simulink model "untitled2"  (R2024b)
settings: Solver=FixedStepAuto  StartTime=0.0  StopTime=inf  FixedStep=0.01  RelTol=1e-3  EnableMultiTasking=on
undefined symbols (not defined in the file or in its folder): qbreak
libraries: simulink x70, arduinolib x31, dspswit3 x9, dspstat3 x4, arduinosensorlib x2, dspfdesign x2
(part 1 of 3)
settings Model: ExtModeTrigDuration=2  Creator=ARIES  LastModifiedBy=ARIES
settings SolverCC: AutoInsertRateTranBlk=on
settings OptimizationCC: EnhancedBackFolding=on  PassReuseOutputArgsAs=Individual arguments  ZeroExternalMemoryAtStartup=off  ZeroInternalMemoryAtStartup=off  MaxStackSize=64  OptimizeBlockOrder=speed  DifferentSizesBufferReuse=on  OptimizationCustomize=off  EfficientTunableParamExpr=on
settings DebuggingCC: ParameterTunabilityLossMsg=error
settings HardwareCC: ProdBitPerPointer=32  ProdBitPerSizeT=32  ProdBitPerPtrDiffT=32  ProdLargestAtomicInteger=Long  ProdLargestAtomicFloat=Double  ProdWordSize=32  ProdHWDeviceType=ARM Compatible->ARM Cortex
settings SFSimCC: MATLABDynamicMemAlloc=off
settings RTWCC: Description=Embedded Coder  SystemTargetFile=ert.tlc  HardwareBoard=Arduino MKR WiFi 1010  TemplateMakefile=ert_default_tmf  Toolchain=Arduino ARM  BuildConfiguration=Faster Runs
settings CodeAppCC: ForceParamTrailComments=on  IgnoreCustomStorageClasses=off  OperatorAnnotations=on  SimulinkDataObjDesc=on  SFDataObjDesc=on  InsertBlockDesc=on
settings ERTTargetCC: SupportContinuousTime=on  SupportVariableSizeSignals=on  ExtModeTransport=3  ExtModeStaticAlloc=on  ExtModeAutomaticAllocSize=off  ExtModeStaticAllocSize=8192  ExtModeMexFile=ext_xcp  ExtModeIntrfLevel=Level2 - Open  InlinedParameterPlacement=Hierarchical

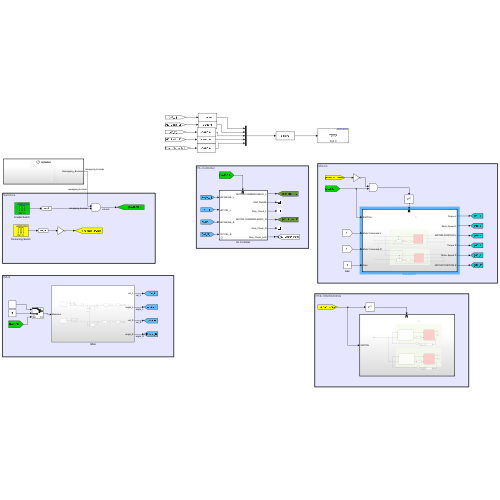
[thumbnail: Simulink's stored preview of the top-level diagram]
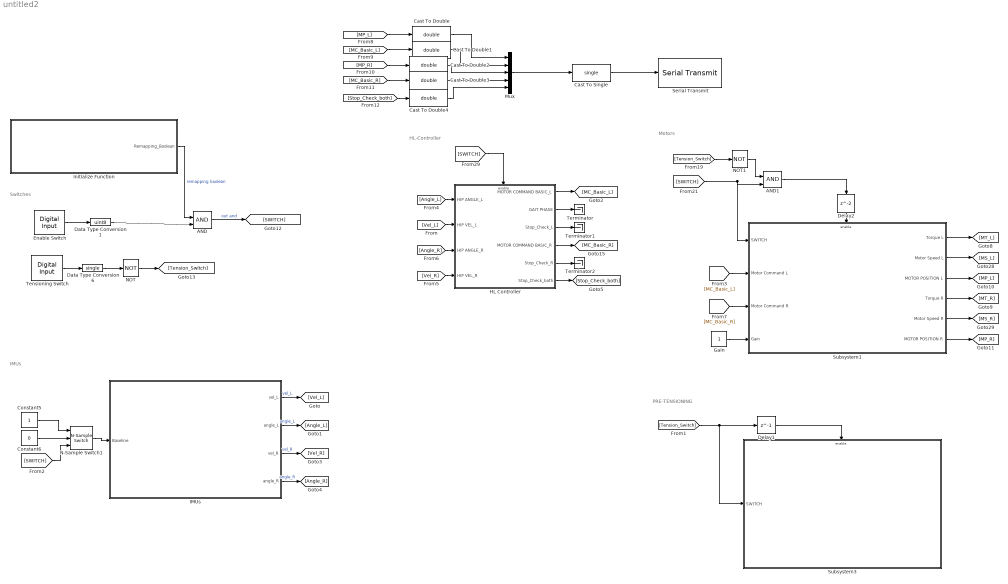
== system untitled2 ==
  note: PRE-TENSIONING
  note: Switches
  note: HL-Controller
  note: IMUs
  note: Motors
  AND : Logic  IconShape=distinctive  AllPortsSameDT=off  OutDataTypeStr=boolean
  AND1 : Logic  IconShape=distinctive  AllPortsSameDT=off  OutDataTypeStr=boolean
  Cast To Double{,1..4} (5 alike) : DataTypeConversion  OutDataTypeStr=double  SaturateOnIntegerOverflow=off  RndMeth=Floor
  Cast To Single : DataTypeConversion  OutDataTypeStr=single  SaturateOnIntegerOverflow=off  RndMeth=Floor
  Constant5 : Constant
  Constant6 : Constant  Value=0
  Data Type Conversion1 : DataTypeConversion  OutDataTypeStr=uint8  SaturateOnIntegerOverflow=off  RndMeth=Floor
  Data Type Conversion6 : DataTypeConversion  OutDataTypeStr=single  SaturateOnIntegerOverflow=off  RndMeth=Floor
  Delay1 : Delay  DelayLength=1
  Delay2 : Delay
  Enable Switch : arduinolib/Digital Input  pinNumber=6  mode=Default  Direction=input  SampleTime=0.01  blockPlatform=arduino
      settings: SourceProductName=Common
  Gain : Constant
  HL Controller : Subsystem  mask{LAG=pi/7, THR=5, AMPL=-6.5}
      mask prompts: LAG "Lag compensation (rad)"; THR "Stop Threshold"; AMPL "Motor position desired amplitude"
  IMUs : Subsystem
  Initialize Function : Subsystem  TreatAsAtomicUnit=on
  Mux : Mux  Inputs=5
  N-Sample Switch1 : dspswit3/N-Sample Switch  N=10  reset=on  TriggerType=Rising edge  Ts=0.01
  NOT : Logic  Operator=NOT  IconShape=distinctive  AllPortsSameDT=off  OutDataTypeStr=boolean
  NOT1 : Logic  Operator=NOT  IconShape=distinctive  AllPortsSameDT=off  OutDataTypeStr=boolean
  Serial Transmit : arduinolib/Serial Transmit  portNumber=0  sendmode=write  sendformat=Decimal  floatprecision=2  header=[]  terminator=[]  blockPlatform=ARDUINO
      settings: SourceProductName=Common
  Subsystem1 : Subsystem
  Subsystem3 : Subsystem
  Tensioning Switch : arduinolib/Digital Input  pinNumber=5  mode=Input Pullup  Direction=input  SampleTime=0.01  blockPlatform=arduino
      settings: SourceProductName=Common
  Terminator : Terminator
  Terminator1 : Terminator
  Terminator2 : Terminator
  wires:
  Subsystem1/1(Torque L) -> [MT_L]
  AND/1 -> [SWITCH]  "out and"
  [Tension_Switch] -> NOT1/1
  IMUs/4(angle_R) -> [Angle_R]  "angle_R"
  Tensioning Switch/1 -> Data Type Conversion6/1
  Subsystem1/6(MOTOR POSITION R) -> [MP_R]
  Constant5/1 -> N-Sample Switch1/1
  [Tension_Switch] -> Subsystem3/1(SWITCH), Delay1/1
  IMUs/3(vel_R) -> [Vel_R]  "vel_R"
  AND1/1 -> Delay2/1
  NOT1/1 -> AND1/1
  Subsystem1/3(MOTOR POSITION L) -> [MP_L]
  Data Type Conversion6/1 -> NOT/1
  [Vel_R] -> HL Controller/4(HIP VEL_R)
  HL Controller/1(MOTOR COMMAND BASIC_L) -> [MC_Basic_L]
  Delay2/1 -> Subsystem1/Enable
  HL Controller/4(MOTOR COMMAND BASIC_R) -> [MC_Basic_R]
  Enable Switch/1 -> Data Type Conversion1/1
  IMUs/2(angle_L) -> [Angle_L]  "angle_L"
  Subsystem1/5(Motor Speed R) -> [MS_R]
  Data Type Conversion1/1 -> AND/2
  N-Sample Switch1/1 -> IMUs/1(Baseline)
  Delay1/1 -> Subsystem3/Enable
  NOT/1 -> [Tension_Switch]
  Constant6/1 -> N-Sample Switch1/2
  [Angle_R] -> HL Controller/3(HIP ANGLE_R)
  Subsystem1/2(Motor Speed L) -> [MS_L]
  [SWITCH] -> HL Controller/Enable
  Initialize Function/1(Remapping_Boolean) -> AND/1  "remapping boolean"
  [MC_Basic_R] -> Subsystem1/3(Motor Command R)
  [SWITCH] -> N-Sample Switch1/3
  [Angle_L] -> HL Controller/1(HIP ANGLE_L)
  [Vel_L] -> HL Controller/2(HIP VEL_L)
  IMUs/1(vel_L) -> [Vel_L]  "vel_L"
  [SWITCH] -> AND1/2, Subsystem1/1(SWITCH)
  Subsystem1/4(Torque R) -> [MT_R]
  [MC_Basic_L] -> Subsystem1/2(Motor Command L)
  Gain/1 -> Subsystem1/4(Gain)
  Mux/1 -> Cast To Single/1
  Cast To Single/1 -> Serial Transmit/1
  [MP_L] -> Cast To Double/1
  [MC_Basic_L] -> Cast To Double1/1
  [MP_R] -> Cast To Double2/1
  [MC_Basic_R] -> Cast To Double3/1
  HL Controller/6(Stop_Check_both) -> [Stop_Check_both]
  [Stop_Check_both] -> Cast To Double4/1
  HL Controller/5(Stop_Check_R) -> Terminator2/1
  HL Controller/3(Stop_Check_L) -> Terminator1/1
  HL Controller/2(GAIT PHASE) -> Terminator/1
  Cast To Double/1 -> Mux/1
  Cast To Double1/1 -> Mux/2
  Cast To Double3/1 -> Mux/4
  Cast To Double2/1 -> Mux/3
  Cast To Double4/1 -> Mux/5

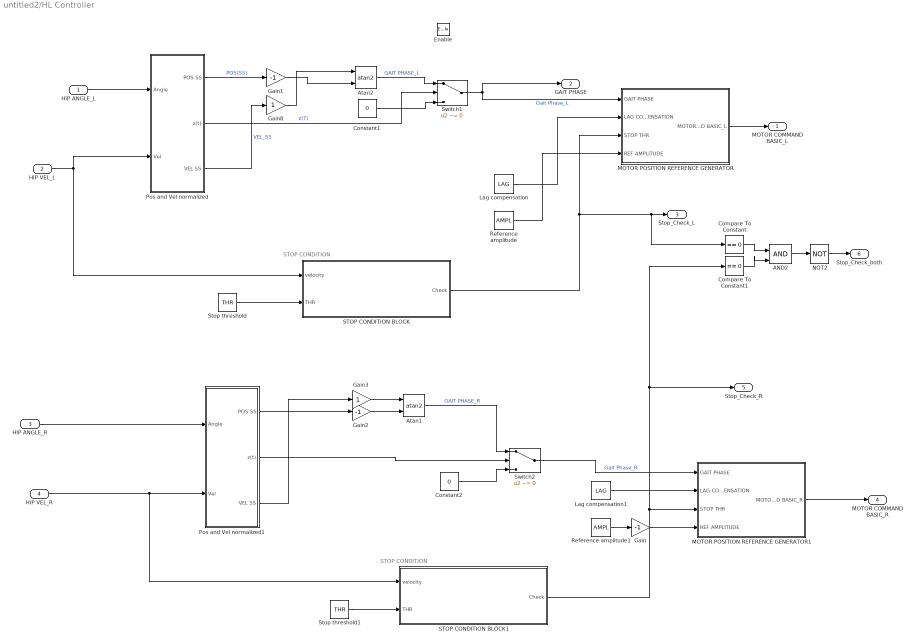
== system untitled2/HL Controller ==
  note: STOP CONDITION
  note: STOP CONDITION
  HIP ANGLE_L : Inport
  HIP VEL_L : Inport  Port=2
  HIP ANGLE_R : Inport  Port=3
  HIP VEL_R : Inport  Port=4
  Enable : EnablePort
  AND2 : Logic  IconShape=distinctive  AllPortsSameDT=off  OutDataTypeStr=boolean
  Atan1 : Trigonometry  Operator=atan2
  Atan2 : Trigonometry  Operator=atan2
  Compare To Constant : simulink/Logic and Bit Operations/Compare To Constant  relop===  const=0  OutDataTypeStr=boolean
  Compare To Constant1 : simulink/Logic and Bit Operations/Compare To Constant  relop===  const=0  OutDataTypeStr=boolean
  Constant1 : Constant  Value=0
  Constant2 : Constant  Value=0
  Gain : Gain  Gain=-1
  Gain1 : Gain  Gain=-1
  Gain2 : Gain  Gain=-1
  Gain3 : Gain
  Gain8 : Gain
  Lag compensation : Constant  Value=LAG
  Lag compensation1 : Constant  Value=LAG
  MOTOR POSITION REFERENCE GENERATOR : Subsystem
  MOTOR POSITION REFERENCE GENERATOR1 : Subsystem
  NOT2 : Logic  Operator=NOT  IconShape=distinctive  AllPortsSameDT=off  OutDataTypeStr=boolean
  Pos and Vel normalized : Subsystem
  Pos and Vel normalized1 : Subsystem
  Reference amplitude : Constant  Value=AMPL
  Reference amplitude1 : Constant  Value=AMPL
  STOP CONDITION BLOCK : Subsystem
  STOP CONDITION BLOCK1 : Subsystem
  Stop threshold : Constant  Value=THR
  Stop threshold1 : Constant  Value=THR
  Switch1 : Switch  Criteria=u2 ~= 0  SaturateOnIntegerOverflow=off  InputSameDT=off
  Switch2 : Switch  Criteria=u2 ~= 0  SaturateOnIntegerOverflow=off  InputSameDT=off
  MOTOR COMMAND BASIC_L : Outport
  GAIT PHASE : Outport  Port=2
  Stop_Check_L : Outport  Port=3
  MOTOR COMMAND BASIC_R : Outport  Port=4
  Stop_Check_R : Outport  Port=5
  Stop_Check_both : Outport  Port=6
  wires:
  Gain8/1 -> Atan2/1
  Atan2/1 -> Switch1/1  "GAIT PHASE_L"
  Switch1/1 -> GAIT PHASE/1, MOTOR POSITION REFERENCE GENERATOR/1(GAIT PHASE)  "Gait Phase_L"
  Constant1/1 -> Switch1/3
  Gain1/1 -> Atan2/2
  Pos and Vel normalized/1(POS SS) -> Gain1/1  "POS(SS)"
  Pos and Vel normalized/2(z(t)) -> Switch1/2  "z(T)"
  Pos and Vel normalized/3(VEL SS) -> Gain8/1  "VEL_SS"
  HIP VEL_L/1 -> STOP CONDITION BLOCK/1(velocity), Pos and Vel normalized/2(Vel)
  HIP ANGLE_L/1 -> Pos and Vel normalized/1(Angle)
  Lag compensation/1 -> MOTOR POSITION REFERENCE GENERATOR/2(LAG COMPENSATION)
  Stop threshold/1 -> STOP CONDITION BLOCK/2(THR)
  Reference amplitude/1 -> MOTOR POSITION REFERENCE GENERATOR/4(REF AMPLITUDE)
  MOTOR POSITION REFERENCE GENERATOR/1(MOTOR COMMAND BASIC_L) -> MOTOR COMMAND BASIC_L/1
  Switch2/1 -> MOTOR POSITION REFERENCE GENERATOR1/1(GAIT PHASE)  "Gait Phase_R"
  Lag compensation1/1 -> MOTOR POSITION REFERENCE GENERATOR1/2(LAG COMPENSATION)
  Stop threshold1/1 -> STOP CONDITION BLOCK1/2(THR)
  Pos and Vel normalized1/2(z(t)) -> Switch2/2
  Pos and Vel normalized1/1(POS SS) -> Gain2/1
  Gain2/1 -> Atan1/2
  Constant2/1 -> Switch2/3
  Gain3/1 -> Atan1/1
  Pos and Vel normalized1/3(VEL SS) -> Gain3/1
  Atan1/1 -> Switch2/1  "GAIT PHASE_R"
  HIP ANGLE_R/1 -> Pos and Vel normalized1/1(Angle)
  MOTOR POSITION REFERENCE GENERATOR1/1(MOTOR COMMAND BASIC_R) -> MOTOR COMMAND BASIC_R/1
  HIP VEL_R/1 -> STOP CONDITION BLOCK1/1(velocity), Pos and Vel normalized1/2(Vel)
  Reference amplitude1/1 -> Gain/1
  Compare To Constant1/1 -> AND2/2
  NOT2/1 -> Stop_Check_both/1
  AND2/1 -> NOT2/1
  STOP CONDITION BLOCK1/1(Check) -> MOTOR POSITION REFERENCE GENERATOR1/3(STOP THR), Stop_Check_R/1, Compare To Constant1/1
  Compare To Constant/1 -> AND2/1
  STOP CONDITION BLOCK/1(Check) -> MOTOR POSITION REFERENCE GENERATOR/3(STOP THR), Stop_Check_L/1, Compare To Constant/1
  Gain/1 -> MOTOR POSITION REFERENCE GENERATOR1/4(REF AMPLITUDE)

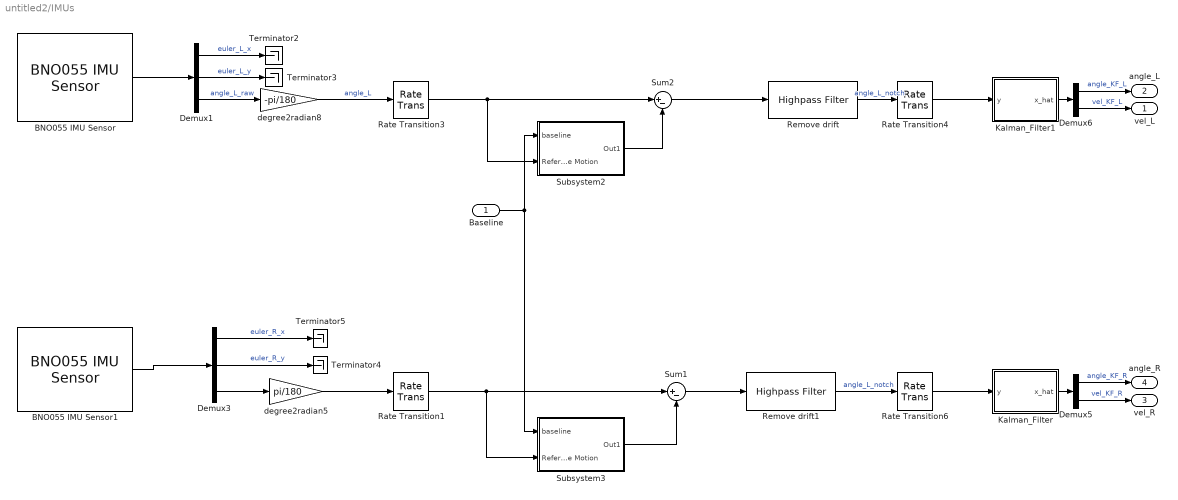
== system untitled2/IMUs ==
  Baseline : Inport
  BNO055 IMU Sensor : arduinosensorlib/BNO055 IMU Sensor  I2CModule=0  SlaveAddress=0x28  OperationMode=Fusion  Accel=off  AngularRate=off  MagField=off  EulerAngles=on  Quat=off  LinearAccel=off  GravityVector=off  Status=off  Timestamp=off  AccelRange=4G  AccelBW=62.5 Hz  GyroRange=2000 dps  GyroBW=32 Hz  MagODR=10 Hz  spf=1  SampleTime=-1  blockPlatform=ARDUINO  QueueSizeFactor=1
      settings: SourceProductName=Sensors
  BNO055 IMU Sensor1 : arduinosensorlib/BNO055 IMU Sensor  I2CModule=0  SlaveAddress=0x29  OperationMode=Fusion  Accel=off  AngularRate=off  MagField=off  EulerAngles=on  Quat=off  LinearAccel=off  GravityVector=off  Status=off  Timestamp=off  AccelRange=4G  AccelBW=62.5 Hz  GyroRange=2000 dps  GyroBW=32 Hz  MagODR=10 Hz  spf=1  SampleTime=-1  blockPlatform=ARDUINO  QueueSizeFactor=1
      settings: SourceProductName=Sensors
  Demux1 : Demux  Outputs=3
  Demux3 : Demux  Outputs=3
  Demux5 : Demux  Outputs=2
  Demux6 : Demux  Outputs=2
  Kalman_Filter : MATLAB Function  TreatAsAtomicUnit=on
  Kalman_Filter1 : MATLAB Function  TreatAsAtomicUnit=on
  Rate Transition{1,3..4,6} (4 alike) : RateTransition  OutPortSampleTime=0.01
  Remove drift : dspfdesign/Highpass Filter  FilterType=IIR  DesignForMinimumOrder=off  FilterOrder=2  StopbandFrequency=8e3  PassbandFrequency=0.1  StopbandAttenuation=40  PassbandRipple=0.1  SampleRateMode=Specify on dialog  SampleRate=100  SimulateUsing=Interpreted execution  roundingMode=Floor  coeffsDataTypeStr=fixdt(1,16)
  Remove drift1 : dspfdesign/Highpass Filter  FilterType=IIR  DesignForMinimumOrder=off  FilterOrder=2  StopbandFrequency=8e3  PassbandFrequency=0.1  StopbandAttenuation=40  PassbandRipple=0.1  SampleRateMode=Specify on dialog  SampleRate=100  SimulateUsing=Interpreted execution  roundingMode=Floor  coeffsDataTypeStr=fixdt(1,16)
  Subsystem2 : Subsystem
  Subsystem3 : Subsystem
  Sum1 : Sum  Inputs=|+-
  Sum2 : Sum  Inputs=|+-
  Terminator{2..5} (4 alike) : Terminator
  degree2radian5 : Gain  Gain=pi/180
  degree2radian8 : Gain  Gain=-pi/180
  vel_L : Outport
  angle_L : Outport  Port=2
  vel_R : Outport  Port=3
  angle_R : Outport  Port=4
  wires:
  BNO055 IMU Sensor/1 -> Demux1/1
  BNO055 IMU Sensor1/1 -> Demux3/1
  Demux1/1 -> Terminator2/1  "euler_L_x"
  Demux1/3 -> degree2radian8/1  "angle_L_raw"
  Demux1/2 -> Terminator3/1  "euler_L_y"
  Demux3/1 -> Terminator5/1  "euler_R_x"
  Demux3/2 -> Terminator4/1  "euler_R_y"
  Demux3/3 -> degree2radian5/1
  Remove drift/1 -> Rate Transition4/1  "angle_L_notch"
  Remove drift1/1 -> Rate Transition6/1  "angle_L_notch"
  Kalman_Filter/1(x_hat) -> Demux5/1
  Demux5/1 -> angle_R/1  "angle_KF_R"
  Demux5/2 -> vel_R/1  "vel_KF_R"
  Sum2/1 -> Remove drift/1
  Rate Transition3/1 -> Subsystem2/2(Reference Motion), Sum2/1
  Baseline/1 -> Subsystem2/1(baseline), Subsystem3/1(baseline)
  Subsystem2/1(Out1) -> Sum2/2
  Rate Transition1/1 -> Subsystem3/2(Reference Motion), Sum1/1
  Subsystem3/1(Out1) -> Sum1/2
  Sum1/1 -> Remove drift1/1
  degree2radian8/1 -> Rate Transition3/1  "angle_L"
  degree2radian5/1 -> Rate Transition1/1
  Rate Transition6/1 -> Kalman_Filter/1(y)
  Demux6/1 -> angle_L/1  "angle_KF_L"
  Demux6/2 -> vel_L/1  "vel_KF_L"
  Kalman_Filter1/1(x_hat) -> Demux6/1
  Rate Transition4/1 -> Kalman_Filter1/1(y)

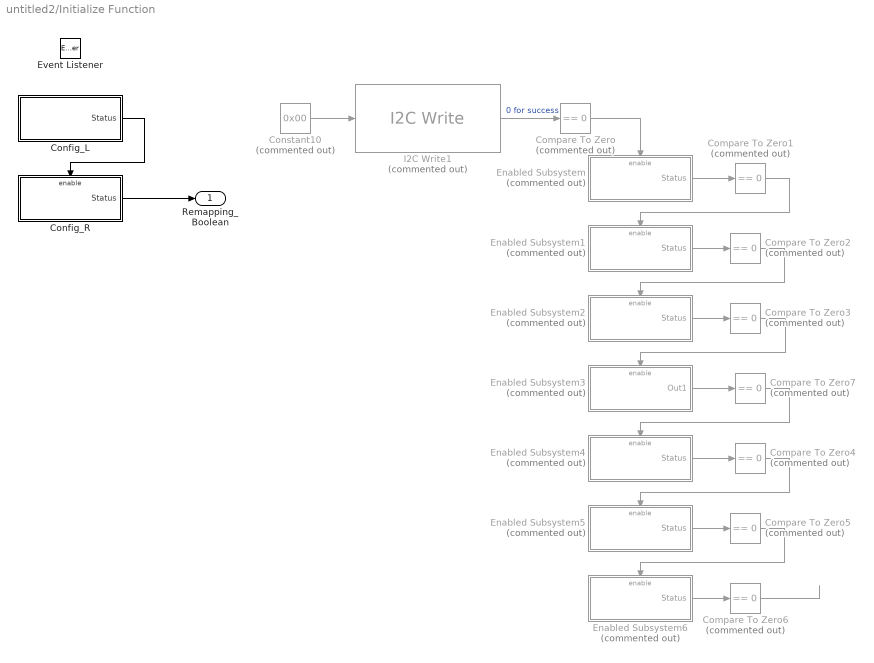
== system untitled2/Initialize Function ==
  Compare To Zero{,1..7} (8 alike) : simulink/Logic and Bit Operations/Compare To Zero  Commented=on  relop===  OutDataTypeStr=boolean
  "Config_L " : Subsystem  TreatAsAtomicUnit=on
  Config_R : Subsystem  TreatAsAtomicUnit=on
  Constant10 : Constant  Commented=on  Value=0x00
  Enabled Subsystem : Subsystem  Commented=on  TreatAsAtomicUnit=on
  Enabled Subsystem1 : Subsystem  Commented=on  TreatAsAtomicUnit=on
  Enabled Subsystem2 : Subsystem  Commented=on  TreatAsAtomicUnit=on
  Enabled Subsystem3 : Subsystem  Commented=on  TreatAsAtomicUnit=on
  Enabled Subsystem4 : Subsystem  Commented=on  TreatAsAtomicUnit=on
  Enabled Subsystem5 : Subsystem  Commented=on  TreatAsAtomicUnit=on
  Enabled Subsystem6 : Subsystem  Commented=on  TreatAsAtomicUnit=on
  Event Listener : EventListener  DisableCoverage=on  EventName=reset
  I2C Write1 : arduinolib/I2C Write  Commented=on  I2CModule=0  Mode=Master  SlaveAddress=0x29  SlaveByteOrder=BigEndian  Direction=Transmitter  RegisterAddressMode=on  RegisterAddress=0x3D  SlaveDataType=uint8  DataLength=1  NoAck=off  RepeatedStart=off  OutputStatus=on  blockPlatform=ARDUINO
      settings: SourceProductName=Common
  Remapping_Boolean : Outport
  wires:
  Compare To Zero/1 -> Enabled Subsystem/Enable
  I2C Write1/1 -> Compare To Zero/1  "0 for success"
  Constant10/1 -> I2C Write1/1
  Enabled Subsystem/1(Status) -> Compare To Zero1/1
  Compare To Zero1/1 -> Enabled Subsystem1/Enable
  Enabled Subsystem1/1(Status) -> Compare To Zero2/1
  Compare To Zero2/1 -> Enabled Subsystem2/Enable
  Enabled Subsystem2/1(Status) -> Compare To Zero3/1
  Compare To Zero3/1 -> Enabled Subsystem3/Enable
  Enabled Subsystem5/1(Status) -> Compare To Zero5/1
  Enabled Subsystem6/1(Status) -> Compare To Zero6/1
  Compare To Zero4/1 -> Enabled Subsystem5/Enable
  Enabled Subsystem4/1(Status) -> Compare To Zero4/1
  Compare To Zero5/1 -> Enabled Subsystem6/Enable
  Enabled Subsystem3/1(Out1) -> Compare To Zero7/1
  Compare To Zero7/1 -> Enabled Subsystem4/Enable
  Compare To Zero6/1 -> ?
  "Config_L "/1(Status) -> Config_R/Enable
  Config_R/1(Status) -> Remapping_Boolean/1

== system untitled2/Subsystem1 ==
  note: LeftLeg_AK60-6 Motor Modules
  note: RightLeg_AK60-6 Motor Modules
  SWITCH : Inport
  Motor Command L : Inport  Port=2
  Motor Command R : Inport  Port=3
  Gain : Inport  Port=4
  Enable : EnablePort  StatesWhenEnabling=reset
  Data Type Conversion1 : DataTypeConversion  OutDataTypeStr=single  SaturateOnIntegerOverflow=off  RndMeth=Floor
  Data Type Conversion2 : DataTypeConversion  OutDataTypeStr=single  SaturateOnIntegerOverflow=off  RndMeth=Floor
  Left Motor Velocity1 : Subsystem
  PID1 : Subsystem
  PID2 : Subsystem
  Product : Product
  Product1 : Product
  Right Motor Velocity1 : Subsystem
  Torque L : Outport
  Motor Speed L : Outport  Port=2
  MOTOR POSITION L : Outport  Port=3
  Torque R : Outport  Port=4
  Motor Speed R : Outport  Port=5
  MOTOR POSITION R : Outport  Port=6
  wires:
  Motor Command L/1 -> PID1/1(Ref)
  PID1/1(Velocity output) -> Product/1
  Left Motor Velocity1/1(MOTOR POSITION) -> PID1/2(Actual Motion), MOTOR POSITION L/1
  Data Type Conversion1/1 -> Left Motor Velocity1/2(Motor command)
  Motor Command R/1 -> PID2/1(Ref)
  PID2/1(Velocity output) -> Product1/2
  SWITCH/1 -> PID2/Enable, Right Motor Velocity1/1(SWITCH), Left Motor Velocity1/1(SWITCH), PID1/Enable
  Data Type Conversion2/1 -> Right Motor Velocity1/2(Motor command)
  Left Motor Velocity1/3(MOTOR TORQUE) -> Torque L/1
  Left Motor Velocity1/2(MOTOR SPEED) -> Motor Speed L/1
  Right Motor Velocity1/1(MOTOR POSITION) -> MOTOR POSITION R/1, PID2/2(Actual Motion)
  Right Motor Velocity1/2(MOTOR SPEED) -> Motor Speed R/1
  Right Motor Velocity1/3(MOTOR TORQUE) -> Torque R/1
  Product/1 -> Data Type Conversion1/1
  Product1/1 -> Data Type Conversion2/1
  Gain/1 -> Product1/1, Product/2

== system untitled2/Subsystem3 ==
  note: RightLeg_AK60-6 Motor Modules
  note: LeftLeg_AK60-6 Motor Modules
  SWITCH : Inport
  Enable : EnablePort  StatesWhenEnabling=reset
  Abs : Abs  SaturateOnIntegerOverflow=off
  Abs1 : Abs  SaturateOnIntegerOverflow=off
  Chart : Stateflow chart  TreatAsAtomicUnit=on
  Chart1 : Stateflow chart  TreatAsAtomicUnit=on
  Data Type Conversion1 : DataTypeConversion  OutDataTypeStr=single  SaturateOnIntegerOverflow=off  RndMeth=Floor
  Data Type Conversion6 : DataTypeConversion  OutDataTypeStr=single  SaturateOnIntegerOverflow=off  RndMeth=Floor
  Left Motor Velocity : Subsystem
  Right Motor Velocity : Subsystem
  Subsystem1 : Subsystem  mask{wn=25, zt=1, x0=0}
      mask prompts: wn "Cut-off frequency (rad/s)"; zt "Damping ratio"; x0 "Initial Condition"
      mask Display: disp('Second-Order\nLow-Pass Filter');
  Subsystem4 : Subsystem  mask{wn=25, zt=1, x0=0}
      mask prompts: wn "Cut-off frequency (rad/s)"; zt "Damping ratio"; x0 "Initial Condition"
      mask Display: disp('Second-Order\nLow-Pass Filter');
  Terminator{1..6} (6 alike) : Terminator
  wires:
  Chart1/2(vel) -> Data Type Conversion1/1
  SWITCH/1 -> Chart1/2(ON_OFF), Chart/2(ON_OFF)
  Data Type Conversion6/1 -> Right Motor Velocity/2(Motor command)
  Left Motor Velocity/3(MOTOR TORQUE) -> Subsystem1/1(x)
  Right Motor Velocity/2(MOTOR SPEED) -> Terminator2/1
  Left Motor Velocity/2(MOTOR SPEED) -> Terminator1/1
  Chart/2(vel) -> Data Type Conversion6/1
  Right Motor Velocity/1(MOTOR POSITION) -> Terminator4/1
  Subsystem4/1(y) -> Abs/1  "TORQUE"
  Right Motor Velocity/3(MOTOR TORQUE) -> Subsystem4/1(x)
  Subsystem4/2(yd) -> Terminator5/1
  Abs/1 -> Chart/1(MOTOR_TORQUE)
  Left Motor Velocity/1(MOTOR POSITION) -> Terminator3/1
  Subsystem1/1(y) -> Abs1/1  "TORQUE"
  Subsystem1/2(yd) -> Terminator6/1
  Abs1/1 -> Chart1/1(MOTOR_TORQUE)
  Chart/1(enablestati) -> Right Motor Velocity/1(SWITCH)
  Chart1/1(enablestati) -> Left Motor Velocity/1(SWITCH)
  Data Type Conversion1/1 -> Left Motor Velocity/2(Motor command)

== system untitled2/HL Controller/MOTOR POSITION REFERENCE GENERATOR ==
  note: KALMAN FILTER
  GAIT PHASE : Inport
  LAG COMPENSATION : Inport  Port=2
  STOP THR : Inport  Port=3
  REF AMPLITUDE : Inport  Port=4
  Demux : Demux  Outputs=2
  Gain : Gain  Gain=-1
  Motion mapping2 : Lookup_n-D  NumberOfTableDimensions=1  BreakpointsForDimension1=[-1, -0.8, -0.6, -0.4, -0.2, -0.1, 0, 0.1, 0.2, 0.4, 0.6, 0.8, 1]  BreakpointsForDimension2=qbreak(:,2)  Table=[-1, -0.8, -0.6, -0.4, -0.2, -0.1, 0, 0, 0.005, 0.01, 0.015,0.02,0.025]  InterpMethod=Cubic spline  ExtrapMethod=Cubic spline  InternalRulePriority=Speed  RndMeth=Simplest
  Plus : Sum
  Product : Product
  Rate Transition : RateTransition
  Ref traj w/ noise : MATLAB Function  TreatAsAtomicUnit=on
  Saturation : Saturate  UpperLimit=600*pi/180  LowerLimit=-600*pi/180
  Sin1 : Trigonometry
  Switch3 : Switch  Criteria=u2 > Threshold  SaturateOnIntegerOverflow=off  InputSameDT=off
  Terminator : Terminator
  MOTOR COMMAND BASIC_L : Outport
  wires:
  Ref traj w/ noise/1(x_hat) -> Demux/1
  Demux/2 -> Terminator/1
  Motion mapping2/1 -> Product/1
  STOP THR/1 -> Switch3/2, Switch3/3
  Switch3/1 -> Rate Transition/1
  Product/1 -> Saturation/1
  Sin1/1 -> Gain/1
  Plus/1 -> Sin1/1
  Demux/1 -> Motion mapping2/1
  Rate Transition/1 -> Ref traj w/ noise/1(y)
  Saturation/1 -> MOTOR COMMAND BASIC_L/1
  GAIT PHASE/1 -> Plus/1
  LAG COMPENSATION/1 -> Plus/2
  REF AMPLITUDE/1 -> Product/2
  Gain/1 -> Switch3/1

== system untitled2/HL Controller/MOTOR POSITION REFERENCE GENERATOR1 ==
  note: KALMAN FILTER
  GAIT PHASE : Inport
  LAG COMPENSATION : Inport  Port=2
  STOP THR : Inport  Port=3
  REF AMPLITUDE : Inport  Port=4
  Demux : Demux  Outputs=2
  Gain : Gain  Gain=-1
  Motion mapping2 : Lookup_n-D  NumberOfTableDimensions=1  BreakpointsForDimension1=[-1, -0.8, -0.6, -0.4, -0.2, -0.1, 0, 0.1, 0.2, 0.4, 0.6, 0.8, 1]  BreakpointsForDimension2=qbreak(:,2)  Table=[-1, -0.8, -0.6, -0.4, -0.2, -0.1, 0, 0, 0.005, 0.01, 0.015,0.02,0.025]  InterpMethod=Cubic spline  ExtrapMethod=Cubic spline  InternalRulePriority=Speed  RndMeth=Simplest
  Plus : Sum
  Product : Product
  Rate Transition : RateTransition
  Ref traj w/ noise : MATLAB Function  TreatAsAtomicUnit=on
  Saturation : Saturate  UpperLimit=600*pi/180  LowerLimit=-600*pi/180
  Sin1 : Trigonometry
  Switch3 : Switch  Criteria=u2 > Threshold  SaturateOnIntegerOverflow=off  InputSameDT=off
  Terminator : Terminator
  MOTOR COMMAND BASIC_R : Outport
  wires:
  Ref traj w/ noise/1(x_hat) -> Demux/1
  Demux/2 -> Terminator/1
  Motion mapping2/1 -> Product/1
  STOP THR/1 -> Switch3/2, Switch3/3
  Switch3/1 -> Rate Transition/1
  Product/1 -> Saturation/1
  Sin1/1 -> Gain/1
  Plus/1 -> Sin1/1
  Demux/1 -> Motion mapping2/1
  Rate Transition/1 -> Ref traj w/ noise/1(y)
  Saturation/1 -> MOTOR COMMAND BASIC_R/1
  GAIT PHASE/1 -> Plus/1
  LAG COMPENSATION/1 -> Plus/2
  REF AMPLITUDE/1 -> Product/2
  Gain/1 -> Switch3/1

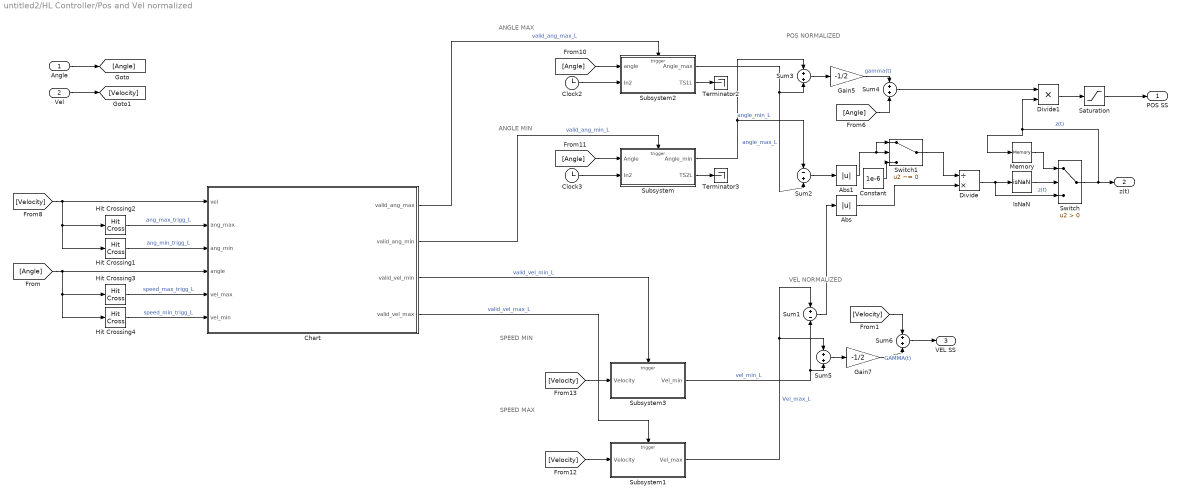
== system untitled2/HL Controller/Pos and Vel normalized ==
  note: ANGLE MIN
  note: ANGLE MAX
  note: SPEED MAX
  note: SPEED MIN
  note: POS NORMALIZED
  note: VEL NORMALIZED
  Angle : Inport
  Vel : Inport  Port=2
  Abs : Abs  SaturateOnIntegerOverflow=off
  Abs1 : Abs  SaturateOnIntegerOverflow=off
  Chart : Stateflow chart  TreatAsAtomicUnit=on
      settings: PortSchema="{\"entries\":[{\"content\":{\"sides\":[{\"content\":{\"connectorIds\":[\"In5\",\"In1\",\"In4\",\"In6\",\"In3\",\"In2\"]},\"type\":\"ConnectorPlacement.EquallySpacedRectSide\",\"uuid\":\"1b4e9464-0c1b-4aef-9691-eb83c0a92a72\"},{\"content\":{\"connectorIds\":[\"Out3\",\"Out4\",\"Out2\",\"Out1\"],\"side\":\"RIGHT\"},\"type\":\"ConnectorPlacement.EquallySpacedRectSide\",\"uuid\":\"791196f6-4c97-40a1-8015-a03f83b94293\"},{\"content\":{\"side\":\"TOP\"},\"type\":\"ConnectorPlacement.EquallySpacedRectSide\",\"uuid\":\"116d3fb6-be2c-4be4-86cc-df9779b501c6\"}]},\"type\":\"ConnectorPlacement.EquallySpacedConnector\",\"uuid\":\"13d090b2-a2d1-429a-b321-7320a6f027c7\"}],\"packageUris\":[\"http://schema.mathworks.com/mf0/Connector/R2020b\"],\"version\":\"1.0\"}"
  Clock2 : Clock
  Clock3 : Clock
  Constant : Constant  Value=1e-6
  Divide : Product  Inputs=/*
  Divide1 : Product  Inputs=**
  Gain5 : Gain  Gain=-1/2
  Gain7 : Gain  Gain=-1/2
  Hit Crossing1 : HitCross  HitCrossingDirection=rising
  Hit Crossing2 : HitCross  HitCrossingDirection=falling
  Hit Crossing3 : HitCross  HitCrossingDirection=rising
  Hit Crossing4 : HitCross  HitCrossingDirection=falling
  IsNaN : RelationalOperator  Operator=isNaN  OutDataTypeStr=boolean  RndMeth=Simplest  InputSameDT=off
  Memory : Memory
  Saturation : Saturate  UpperLimit=10  LowerLimit=-10
  Subsystem : Subsystem
  Subsystem1 : Subsystem
  Subsystem2 : Subsystem
  Subsystem3 : Subsystem
  Sum1 : Sum  Inputs=+-
  Sum2 : Sum  Inputs=-+
  Sum{3..6} (4 alike) : Sum
  Switch : Switch  Criteria=u2 > Threshold  SaturateOnIntegerOverflow=off  InputSameDT=off
  Switch1 : Switch  Criteria=u2 ~= 0  SaturateOnIntegerOverflow=off  InputSameDT=off
  Terminator2 : Terminator
  Terminator3 : Terminator
  POS SS : Outport
  z(t) : Outport  Port=2
  VEL SS : Outport  Port=3
  wires:
  Hit Crossing2/1 -> Chart/1(ang_max)  "ang_max_trigg_L"
  Subsystem2/1(Angle_max) -> Sum2/2, Sum3/2  "angle_max_L"
  Sum4/1 -> Divide1/1
  Sum3/1 -> Gain5/1
  Subsystem/1(Angle_min) -> Sum2/1, Sum3/1  "angle_min_L"
  Hit Crossing1/1 -> Chart/4(ang_min)  "ang_min_trigg_L"
  Sum2/1 -> Abs1/1
  Sum1/1 -> Abs/1
  Gain5/1 -> Sum4/1  "gamma(t)"
  Abs/1 -> Divide/2
  Divide/1 -> IsNaN/1, Switch/3  "z(t)"
  Memory/1 -> Switch/1
  IsNaN/1 -> Switch/2
  Switch/1 -> Memory/1, Divide1/2, z(t)/1  "z(t)"
  Divide1/1 -> Saturation/1
  Saturation/1 -> POS SS/1
  Constant/1 -> Switch1/3
  Abs1/1 -> Switch1/2, Switch1/1
  Switch1/1 -> Divide/1
  Hit Crossing4/1 -> Chart/2(vel_min)  "speed_min_trigg_L"
  Subsystem3/1(Vel_min) -> Sum1/2, Sum5/2  "vel_min_L"
  Subsystem1/1(Vel_max) -> Sum1/1, Sum5/1  "Vel_max_L"
  Sum5/1 -> Gain7/1
  Hit Crossing3/1 -> Chart/3(vel_max)  "speed_max_trigg_L"
  Sum6/1 -> VEL SS/1
  Gain7/1 -> Sum6/2  "GAMMA(t)"
  [Velocity] -> Sum6/1
  Chart/1(valid_vel_max) -> Subsystem1/Trigger  "valid_vel_max_L"
  Chart/4(valid_ang_min) -> Subsystem/Trigger  "valid_ang_min_L"
  Chart/3(valid_ang_max) -> Subsystem2/Trigger  "valid_ang_max_L"
  Chart/2(valid_vel_min) -> Subsystem3/Trigger  "valid_vel_min_L"
  Vel/1 -> [Velocity]
  Angle/1 -> [Angle]
  [Angle] -> Hit Crossing4/1, Hit Crossing3/1, Chart/6(angle)
  [Angle] -> Subsystem/1(Angle)
  [Angle] -> Subsystem2/1(angle)
  [Velocity] -> Subsystem1/1(Velocity)
  [Velocity] -> Subsystem3/1(Velocity)
  [Velocity] -> Hit Crossing1/1, Hit Crossing2/1, Chart/5(vel)
  [Angle] -> Sum4/2
  Clock2/1 -> Subsystem2/2(In2)
  Clock3/1 -> Subsystem/2(In2)
  Subsystem/2(TS2L) -> Terminator3/1
  Subsystem2/2(TS1L) -> Terminator2/1

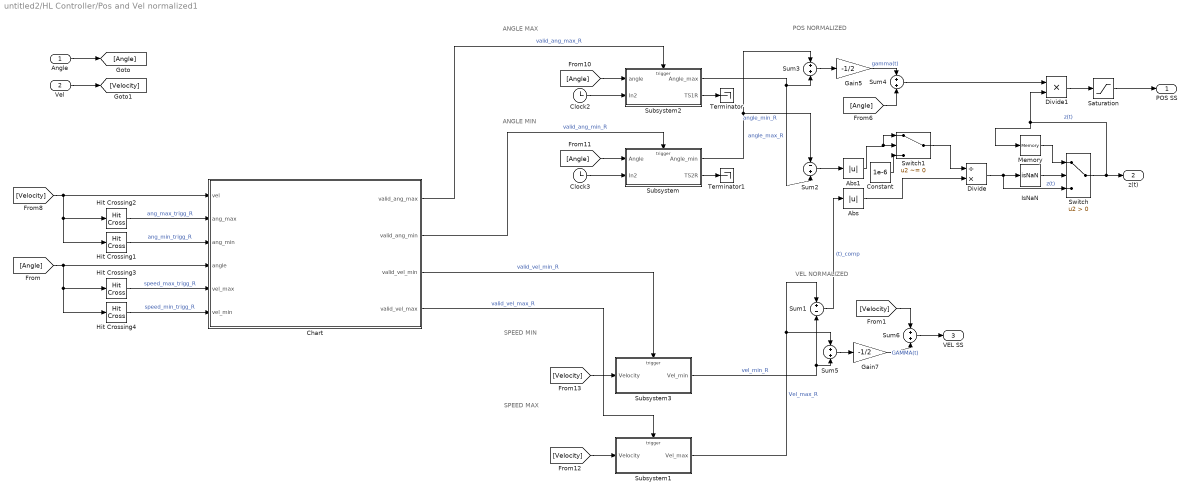
== system untitled2/HL Controller/Pos and Vel normalized1 ==
  note: ANGLE MIN
  note: ANGLE MAX
  note: SPEED MAX
  note: SPEED MIN
  note: POS NORMALIZED
  note: VEL NORMALIZED
  Angle : Inport
  Vel : Inport  Port=2
  Abs : Abs  SaturateOnIntegerOverflow=off
  Abs1 : Abs  SaturateOnIntegerOverflow=off
  Chart : Stateflow chart  TreatAsAtomicUnit=on
      settings: PortSchema="{\"entries\":[{\"content\":{\"sides\":[{\"content\":{\"connectorIds\":[\"In5\",\"In1\",\"In4\",\"In6\",\"In3\",\"In2\"]},\"type\":\"ConnectorPlacement.EquallySpacedRectSide\",\"uuid\":\"1b4e9464-0c1b-4aef-9691-eb83c0a92a72\"},{\"content\":{\"connectorIds\":[\"Out3\",\"Out4\",\"Out2\",\"Out1\"],\"side\":\"RIGHT\"},\"type\":\"ConnectorPlacement.EquallySpacedRectSide\",\"uuid\":\"791196f6-4c97-40a1-8015-a03f83b94293\"},{\"content\":{\"side\":\"TOP\"},\"type\":\"ConnectorPlacement.EquallySpacedRectSide\",\"uuid\":\"116d3fb6-be2c-4be4-86cc-df9779b501c6\"}]},\"type\":\"ConnectorPlacement.EquallySpacedConnector\",\"uuid\":\"13d090b2-a2d1-429a-b321-7320a6f027c7\"}],\"packageUris\":[\"http://schema.mathworks.com/mf0/Connector/R2020b\"],\"version\":\"1.0\"}"
  Clock2 : Clock
  Clock3 : Clock
  Constant : Constant  Value=1e-6
  Divide : Product  Inputs=/*
  Divide1 : Product  Inputs=**
  Gain5 : Gain  Gain=-1/2
  Gain7 : Gain  Gain=-1/2
  Hit Crossing1 : HitCross  HitCrossingDirection=rising
  Hit Crossing2 : HitCross  HitCrossingDirection=falling
  Hit Crossing3 : HitCross  HitCrossingDirection=rising
  Hit Crossing4 : HitCross  HitCrossingDirection=falling
  IsNaN : RelationalOperator  Operator=isNaN  OutDataTypeStr=boolean  RndMeth=Simplest  InputSameDT=off
  Memory : Memory
  Saturation : Saturate  UpperLimit=10  LowerLimit=-10
  Subsystem : Subsystem
  Subsystem1 : Subsystem
  Subsystem2 : Subsystem
  Subsystem3 : Subsystem
  Sum1 : Sum  Inputs=+-
  Sum2 : Sum  Inputs=-+
  Sum{3..6} (4 alike) : Sum
  Switch : Switch  Criteria=u2 > Threshold  SaturateOnIntegerOverflow=off  InputSameDT=off
  Switch1 : Switch  Criteria=u2 ~= 0  SaturateOnIntegerOverflow=off  InputSameDT=off
  Terminator : Terminator
  Terminator1 : Terminator
  POS SS : Outport
  z(t) : Outport  Port=2
  VEL SS : Outport  Port=3
  wires:
  Hit Crossing2/1 -> Chart/1(ang_max)  "ang_max_trigg_R"
  Subsystem2/1(Angle_max) -> Sum2/2, Sum3/2  "angle_max_R"
  Sum4/1 -> Divide1/1
  Sum3/1 -> Gain5/1
  Subsystem/1(Angle_min) -> Sum2/1, Sum3/1  "angle_min_R"
  Hit Crossing1/1 -> Chart/4(ang_min)  "ang_min_trigg_R"
  Sum2/1 -> Abs1/1
  Sum1/1 -> Abs/1  "(t)_comp"
  Gain5/1 -> Sum4/1  "gamma(t)"
  Abs/1 -> Divide/2
  Divide/1 -> IsNaN/1, Switch/3  "z(t)"
  Memory/1 -> Switch/1
  IsNaN/1 -> Switch/2
  Switch/1 -> Memory/1, Divide1/2, z(t)/1  "z(t)"
  Divide1/1 -> Saturation/1
  Saturation/1 -> POS SS/1
  Constant/1 -> Switch1/3
  Abs1/1 -> Switch1/2, Switch1/1
  Switch1/1 -> Divide/1
  Hit Crossing4/1 -> Chart/2(vel_min)  "speed_min_trigg_R"
  Subsystem3/1(Vel_min) -> Sum1/2, Sum5/2  "vel_min_R"
  Subsystem1/1(Vel_max) -> Sum1/1, Sum5/1  "Vel_max_R"
  Sum5/1 -> Gain7/1
  Hit Crossing3/1 -> Chart/3(vel_max)  "speed_max_trigg_R"
  Sum6/1 -> VEL SS/1
  Gain7/1 -> Sum6/2  "GAMMA(t)"
  [Velocity] -> Sum6/1
  Chart/1(valid_vel_max) -> Subsystem1/Trigger  "valid_vel_max_R"
  Chart/4(valid_ang_min) -> Subsystem/Trigger  "valid_ang_min_R"
  Chart/3(valid_ang_max) -> Subsystem2/Trigger  "valid_ang_max_R"
  Chart/2(valid_vel_min) -> Subsystem3/Trigger  "valid_vel_min_R"
  Vel/1 -> [Velocity]
  Angle/1 -> [Angle]
  [Angle] -> Hit Crossing4/1, Hit Crossing3/1, Chart/6(angle)
  [Angle] -> Subsystem/1(Angle)
  [Angle] -> Subsystem2/1(angle)
  [Velocity] -> Subsystem1/1(Velocity)
  [Velocity] -> Subsystem3/1(Velocity)
  [Velocity] -> Hit Crossing1/1, Hit Crossing2/1, Chart/5(vel)
  [Angle] -> Sum4/2
  Clock2/1 -> Subsystem2/2(In2)
  Clock3/1 -> Subsystem/2(In2)
  Subsystem2/2(TS1R) -> Terminator/1
  Subsystem/2(TS2R) -> Terminator1/1

== system untitled2/HL Controller/STOP CONDITION BLOCK ==
  velocity : Inport
  THR : Inport  Port=2
  Gain : Gain  Gain=5
  LP filter : Subsystem  mask{wn=60, zt=1, x0=0}
      mask prompts: wn "Cut-off frequency (rad/s)"; zt "Damping ratio"; x0 "Initial Condition"
      mask Display: disp('Second-Order\nLow-Pass Filter');
  Moving RMS : dspstat3/Moving RMS  Method=Sliding window  ForgettingFactorPort=off  SpecifyWindowLength=on  WindowLength=100  OverlapLength=99  AllowArbitraryInputLength=off  ForgettingFactor=0.9  SimulateUsing=Code generation
  Moving RMS1 : dspstat3/Moving RMS  Method=Sliding window  ForgettingFactorPort=off  SpecifyWindowLength=on  WindowLength=100  OverlapLength=99  AllowArbitraryInputLength=off  ForgettingFactor=0.9  SimulateUsing=Code generation
  Relational Operator : RelationalOperator  OutDataTypeStr=boolean  RndMeth=Simplest  InputSameDT=off
  Sum : Sum
  Check : Outport
  wires:
  Relational Operator/1 -> Check/1
  velocity/1 -> LP filter/1(x)  "θ_dot"
  Moving RMS1/1 -> Sum/1
  LP filter/1(y) -> Gain/1
  LP filter/2(yd) -> Moving RMS/1  "acceleration"
  Moving RMS/1 -> Sum/2
  Sum/1 -> Relational Operator/1
  Gain/1 -> Moving RMS1/1
  THR/1 -> Relational Operator/2

== system untitled2/HL Controller/STOP CONDITION BLOCK1 ==
  velocity : Inport
  THR : Inport  Port=2
  Gain : Gain  Gain=5
  LP filter : Subsystem  mask{wn=60, zt=1, x0=0}
      mask prompts: wn "Cut-off frequency (rad/s)"; zt "Damping ratio"; x0 "Initial Condition"
      mask Display: disp('Second-Order\nLow-Pass Filter');
  Moving RMS : dspstat3/Moving RMS  Method=Sliding window  ForgettingFactorPort=off  SpecifyWindowLength=on  WindowLength=100  OverlapLength=99  AllowArbitraryInputLength=off  ForgettingFactor=0.9  SimulateUsing=Code generation
  Moving RMS1 : dspstat3/Moving RMS  Method=Sliding window  ForgettingFactorPort=off  SpecifyWindowLength=on  WindowLength=100  OverlapLength=99  AllowArbitraryInputLength=off  ForgettingFactor=0.9  SimulateUsing=Code generation
  Relational Operator : RelationalOperator  OutDataTypeStr=boolean  RndMeth=Simplest  InputSameDT=off
  Sum : Sum
  Check : Outport
  wires:
  Relational Operator/1 -> Check/1
  velocity/1 -> LP filter/1(x)  "θ_dot"
  Moving RMS1/1 -> Sum/1
  LP filter/1(y) -> Gain/1
  LP filter/2(yd) -> Moving RMS/1  "acceleration"
  Moving RMS/1 -> Sum/2
  Sum/1 -> Relational Operator/1
  Gain/1 -> Moving RMS1/1
  THR/1 -> Relational Operator/2

== system untitled2/IMUs/Subsystem2 ==
  baseline : Inport
  Reference Motion : Inport  Port=2
  Delay : Delay
  Memory1 : Memory
  Switch1 : Switch  Criteria=u2 > Threshold  SaturateOnIntegerOverflow=off  InputSameDT=off
  Out1 : Outport
  wires:
  Switch1/1 -> Delay/1, Out1/1
  Memory1/1 -> Switch1/3
  baseline/1 -> Switch1/2
  Reference Motion/1 -> Switch1/1
  Delay/1 -> Memory1/1

== system untitled2/IMUs/Subsystem3 ==
  baseline : Inport
  Reference Motion : Inport  Port=2
  Delay : Delay
  Memory1 : Memory
  Switch1 : Switch  Criteria=u2 > Threshold  SaturateOnIntegerOverflow=off  InputSameDT=off
  Out1 : Outport
  wires:
  Switch1/1 -> Delay/1, Out1/1
  Memory1/1 -> Switch1/3
  baseline/1 -> Switch1/2
  Reference Motion/1 -> Switch1/1
  Delay/1 -> Memory1/1

== system untitled2/Initialize Function/Config_L  ==
  Enter Config Mode : Subsystem
  Start Fused (NDOF) Mode : Subsystem  TreatAsAtomicUnit=on
  "X=Z, Y=Y, Z=X" : Subsystem
  Z = -Z : Subsystem  TreatAsAtomicUnit=on
  Status : Outport
  wires:
  Enter Config Mode/1(Status) -> "X=Z, Y=Y, Z=X"/Enable
  Z = -Z/1(Status) -> Start Fused (NDOF) Mode/Enable
  Start Fused (NDOF) Mode/1(Status) -> Status/1
  "X=Z, Y=Y, Z=X"/1(Status) -> Z = -Z/Enable

== system untitled2/Initialize Function/Config_R ==
  Enable : EnablePort
  Enter Config Mode : Subsystem
  Start Fused (NDOF) Mode : Subsystem  TreatAsAtomicUnit=on
  "X=Z, Y=Y, Z=X" : Subsystem
  Z = -Z : Subsystem  TreatAsAtomicUnit=on
  Status : Outport
  wires:
  Start Fused (NDOF) Mode/1(Status) -> Status/1
  "X=Z, Y=Y, Z=X"/1(Status) -> Z = -Z/Enable
  Z = -Z/1(Status) -> Start Fused (NDOF) Mode/Enable
  Enter Config Mode/1(Status) -> "X=Z, Y=Y, Z=X"/Enable

== system untitled2/Initialize Function/Enabled Subsystem ==
  Enable : EnablePort
  Constant13 : Constant  Value=0x06
  I2C Write2 : arduinolib/I2C Write  I2CModule=0  Mode=Master  SlaveAddress=0x29  SlaveByteOrder=BigEndian  Direction=Transmitter  RegisterAddressMode=on  RegisterAddress=0x41  SlaveDataType=uint8  DataLength=1  NoAck=off  RepeatedStart=off  OutputStatus=on  blockPlatform=ARDUINO
      settings: SourceProductName=Common
  Status : Outport
  wires:
  I2C Write2/1 -> Status/1
  Constant13/1 -> I2C Write2/1

== system untitled2/Initialize Function/Enabled Subsystem1 ==
  Enable : EnablePort
  Constant14 : Constant  Value=0x01
  I2C Write3 : arduinolib/I2C Write  I2CModule=0  Mode=Master  SlaveAddress=0x29  SlaveByteOrder=BigEndian  Direction=Transmitter  RegisterAddressMode=on  RegisterAddress=0x42  SlaveDataType=uint8  DataLength=1  NoAck=off  RepeatedStart=off  OutputStatus=on  blockPlatform=ARDUINO
      settings: SourceProductName=Common
  Status : Outport
  wires:
  I2C Write3/1 -> Status/1
  Constant14/1 -> I2C Write3/1

== system untitled2/Initialize Function/Enabled Subsystem2 ==
  Enable : EnablePort
  Constant16 : Constant  Value=0x0C
  I2C Write4 : arduinolib/I2C Write  I2CModule=0  Mode=Master  SlaveAddress=0x29  SlaveByteOrder=BigEndian  Direction=Transmitter  RegisterAddressMode=on  RegisterAddress=0x3D  SlaveDataType=uint8  DataLength=1  NoAck=off  RepeatedStart=off  OutputStatus=on  blockPlatform=ARDUINO
      settings: SourceProductName=Common
  Status : Outport
  wires:
  Constant16/1 -> I2C Write4/1
  I2C Write4/1 -> Status/1

== system untitled2/Initialize Function/Enabled Subsystem3 ==
  Enable : EnablePort
  Constant10 : Constant  Value=0x00
  I2C Write1 : arduinolib/I2C Write  I2CModule=0  Mode=Master  SlaveAddress=0x28  SlaveByteOrder=BigEndian  Direction=Transmitter  RegisterAddressMode=on  RegisterAddress=0x3D  SlaveDataType=uint8  DataLength=1  NoAck=off  RepeatedStart=off  OutputStatus=on  blockPlatform=ARDUINO
      settings: SourceProductName=Common
  Out1 : Outport
  wires:
  I2C Write1/1 -> Out1/1
  Constant10/1 -> I2C Write1/1

== system untitled2/Initialize Function/Enabled Subsystem4 ==
  Enable : EnablePort
  Constant13 : Constant  Value=0x06
  I2C Write2 : arduinolib/I2C Write  I2CModule=0  Mode=Master  SlaveAddress=0x28  SlaveByteOrder=BigEndian  Direction=Transmitter  RegisterAddressMode=on  RegisterAddress=0x41  SlaveDataType=uint8  DataLength=1  NoAck=off  RepeatedStart=off  OutputStatus=on  blockPlatform=ARDUINO
      settings: SourceProductName=Common
  Status : Outport
  wires:
  I2C Write2/1 -> Status/1
  Constant13/1 -> I2C Write2/1

== system untitled2/Initialize Function/Enabled Subsystem5 ==
  Enable : EnablePort
  Constant14 : Constant  Value=0x01
  I2C Write3 : arduinolib/I2C Write  I2CModule=0  Mode=Master  SlaveAddress=0x28  SlaveByteOrder=BigEndian  Direction=Transmitter  RegisterAddressMode=on  RegisterAddress=0x42  SlaveDataType=uint8  DataLength=1  NoAck=off  RepeatedStart=off  OutputStatus=on  blockPlatform=ARDUINO
      settings: SourceProductName=Common
  Status : Outport
  wires:
  I2C Write3/1 -> Status/1
  Constant14/1 -> I2C Write3/1

== system untitled2/Initialize Function/Enabled Subsystem6 ==
  Enable : EnablePort
  Constant16 : Constant  Value=0x0C
  I2C Write4 : arduinolib/I2C Write  I2CModule=0  Mode=Master  SlaveAddress=0x28  SlaveByteOrder=BigEndian  Direction=Transmitter  RegisterAddressMode=on  RegisterAddress=0x3D  SlaveDataType=uint8  DataLength=1  NoAck=off  RepeatedStart=off  OutputStatus=on  blockPlatform=ARDUINO
      settings: SourceProductName=Common
  Status : Outport
  wires:
  Constant16/1 -> I2C Write4/1
  I2C Write4/1 -> Status/1

== system untitled2/Subsystem1/Left Motor Velocity1 ==
  SWITCH : Inport
  Motor command : Inport  Port=2
  Motor Actual Position Receive : Subsystem  Priority=2
  Subsystem : Subsystem  Priority=1
  MOTOR POSITION : Outport
  MOTOR SPEED : Outport  Port=2
  MOTOR TORQUE : Outport  Port=3
  wires:
  Motor command/1 -> Subsystem/1(Motor command)
  SWITCH/1 -> Motor Actual Position Receive/1(SWITCH), Subsystem/2(SWITCH)
  Motor Actual Position Receive/1(MOTOR POSITION) -> MOTOR POSITION/1
  Motor Actual Position Receive/2(MOTOR SPEED) -> MOTOR SPEED/1
  Motor Actual Position Receive/3(MOTOR TORQUE) -> MOTOR TORQUE/1

== system untitled2/Subsystem1/PID1 ==
  Ref : Inport
  Actual Motion : Inport  Port=2
  Enable : EnablePort  StatesWhenEnabling=reset
  Gain4 : Gain  Gain=14
  Gain7 : Gain  Gain=0.02
  Gain8 : Gain  Gain=0
  Integrator1 : Integrator
  Subsystem2 : Subsystem  mask{wn=20, zt=1, x0=0}
      mask prompts: wn "Cut-off frequency (rad/s)"; zt "Damping ratio"; x0 "Initial Condition"
      mask Display: disp('Second-Order\nLow-Pass Filter');
  Sum : Sum  Inputs=|-+  OutDataTypeStr=double
  Sum5 : Sum  Inputs=|+|+|-
  Terminator2 : Terminator
  Velocity output : Outport
  wires:
  Gain7/1 -> Sum5/3
  Subsystem2/2(yd) -> Gain7/1
  Integrator1/1 -> Gain8/1
  Gain4/1 -> Sum5/1
  Actual Motion/1 -> Sum/1
  Gain8/1 -> Sum5/2
  Subsystem2/1(y) -> Terminator2/1
  Sum/1 -> Integrator1/1, Gain4/1
  Ref/1 -> Sum/2
  Sum5/1 -> Velocity output/1, Subsystem2/1(x)

== system untitled2/Subsystem1/PID2 ==
  Ref : Inport
  Actual Motion : Inport  Port=2
  Enable : EnablePort  StatesWhenEnabling=reset
  Gain4 : Gain  Gain=14
  Gain7 : Gain  Gain=0.02
  Gain8 : Gain  Gain=0
  Integrator1 : Integrator
  Subsystem2 : Subsystem  mask{wn=20, zt=1, x0=0}
      mask prompts: wn "Cut-off frequency (rad/s)"; zt "Damping ratio"; x0 "Initial Condition"
      mask Display: disp('Second-Order\nLow-Pass Filter');
  Sum : Sum  Inputs=|-+  OutDataTypeStr=double
  Sum5 : Sum  Inputs=|+|+|-
  Terminator2 : Terminator
  Velocity output : Outport
  wires:
  Gain7/1 -> Sum5/3
  Subsystem2/2(yd) -> Gain7/1
  Integrator1/1 -> Gain8/1
  Gain4/1 -> Sum5/1
  Actual Motion/1 -> Sum/1
  Gain8/1 -> Sum5/2
  Subsystem2/1(y) -> Terminator2/1
  Sum/1 -> Integrator1/1, Gain4/1
  Ref/1 -> Sum/2
  Sum5/1 -> Velocity output/1, Subsystem2/1(x)

== system untitled2/Subsystem1/Right Motor Velocity1 ==
  SWITCH : Inport
  Motor command : Inport  Port=2
  Motor Actual Position Receive : Subsystem  Priority=4
  Subsystem : Subsystem  Priority=3
  MOTOR POSITION : Outport
  MOTOR SPEED : Outport  Port=2
  MOTOR TORQUE : Outport  Port=3
  wires:
  Motor command/1 -> Subsystem/1(Motor command)
  SWITCH/1 -> Motor Actual Position Receive/1(SWITCH), Subsystem/2(SWITCH)
  Motor Actual Position Receive/1(MOTOR POSITION) -> MOTOR POSITION/1
  Motor Actual Position Receive/2(MOTOR SPEED) -> MOTOR SPEED/1
  Motor Actual Position Receive/3(MOTOR TORQUE) -> MOTOR TORQUE/1

== system untitled2/Subsystem3/Left Motor Velocity ==
  SWITCH : Inport
  Motor command : Inport  Port=2
  Motor Actual Position Receive : Subsystem  Priority=4
  Subsystem : Subsystem  Priority=3
  MOTOR POSITION : Outport
  MOTOR SPEED : Outport  Port=2
  MOTOR TORQUE : Outport  Port=3
  wires:
  Motor command/1 -> Subsystem/1(Motor command)
  SWITCH/1 -> Motor Actual Position Receive/1(SWITCH), Subsystem/2(SWITCH)
  Motor Actual Position Receive/1(MOTOR POSITION) -> MOTOR POSITION/1
  Motor Actual Position Receive/2(MOTOR SPEED) -> MOTOR SPEED/1
  Motor Actual Position Receive/3(MOTOR TORQUE) -> MOTOR TORQUE/1

== system untitled2/Subsystem3/Right Motor Velocity ==
  SWITCH : Inport
  Motor command : Inport  Port=2
  Motor Actual Position Receive : Subsystem  Priority=2
  Subsystem : Subsystem  Priority=1
  MOTOR POSITION : Outport
  MOTOR SPEED : Outport  Port=2
  MOTOR TORQUE : Outport  Port=3
  wires:
  Motor command/1 -> Subsystem/1(Motor command)
  SWITCH/1 -> Motor Actual Position Receive/1(SWITCH), Subsystem/2(SWITCH)
  Motor Actual Position Receive/1(MOTOR POSITION) -> MOTOR POSITION/1
  Motor Actual Position Receive/2(MOTOR SPEED) -> MOTOR SPEED/1
  Motor Actual Position Receive/3(MOTOR TORQUE) -> MOTOR TORQUE/1

== system untitled2/Subsystem3/Subsystem1 ==
  x : Inport
  Constant : Constant  Value=2
  Integrator1 : Integrator  InitialConditionSource=external
  Integrator2 : Integrator
  Product : Product  RndMeth=Zero
  Product1 : Product  RndMeth=Zero
  Product2 : Product  Inputs=3  RndMeth=Zero
  Sum : Sum  Inputs=|+-
  Sum1 : Sum  Inputs=|+-
  wn : Constant  Value=wn
  x0 : Constant  Value=x0
  zt : Constant  Value=zt
  y : Outport  VectorParamsAs1DForOutWhenUnconnected=off
  yd : Outport  Port=2  VectorParamsAs1DForOutWhenUnconnected=off
  wires:
  Sum/1 -> Product/2
  wn/1 -> Product/1, Product1/1
  Sum1/1 -> Sum/1
  x0/1 -> Integrator1/2
  Integrator2/1 -> Product1/2, Product2/1
  Product/1 -> Integrator2/1
  x/1 -> Sum1/1
  Product1/1 -> Integrator1/1, yd/1
  Integrator1/1 -> Sum1/2, y/1
  Product2/1 -> Sum/2
  zt/1 -> Product2/3
  Constant/1 -> Product2/2

== system untitled2/Subsystem3/Subsystem4 ==
  x : Inport
  Constant : Constant  Value=2
  Integrator1 : Integrator  InitialConditionSource=external
  Integrator2 : Integrator
  Product : Product  RndMeth=Zero
  Product1 : Product  RndMeth=Zero
  Product2 : Product  Inputs=3  RndMeth=Zero
  Sum : Sum  Inputs=|+-
  Sum1 : Sum  Inputs=|+-
  wn : Constant  Value=wn
  x0 : Constant  Value=x0
  zt : Constant  Value=zt
  y : Outport  VectorParamsAs1DForOutWhenUnconnected=off
  yd : Outport  Port=2  VectorParamsAs1DForOutWhenUnconnected=off
  wires:
  Sum/1 -> Product/2
  wn/1 -> Product/1, Product1/1
  Sum1/1 -> Sum/1
  x0/1 -> Integrator1/2
  Integrator2/1 -> Product1/2, Product2/1
  Product/1 -> Integrator2/1
  x/1 -> Sum1/1
  Product1/1 -> Integrator1/1, yd/1
  Integrator1/1 -> Sum1/2, y/1
  Product2/1 -> Sum/2
  zt/1 -> Product2/3
  Constant/1 -> Product2/2

== system untitled2/HL Controller/Pos and Vel normalized/Subsystem ==
  Angle : Inport
  In2 : Inport  Port=2
  Trigger : TriggerPort  VariantControl=Variant  PortDimensions=1
  Angle_min : Outport
  TS2L : Outport  Port=2
  wires:
  Angle/1 -> Angle_min/1
  In2/1 -> TS2L/1

== system untitled2/HL Controller/Pos and Vel normalized/Subsystem1 ==
  Velocity : Inport
  Trigger : TriggerPort  VariantControl=Variant  PortDimensions=1
  Vel_max : Outport
  wires:
  Velocity/1 -> Vel_max/1

== system untitled2/HL Controller/Pos and Vel normalized/Subsystem2 ==
  angle : Inport
  In2 : Inport  Port=2
  Trigger : TriggerPort  VariantControl=Variant  PortDimensions=1
  Angle_max : Outport
  TS1L : Outport  Port=2
  wires:
  angle/1 -> Angle_max/1
  In2/1 -> TS1L/1

== system untitled2/HL Controller/Pos and Vel normalized/Subsystem3 ==
  Velocity : Inport
  Trigger : TriggerPort  VariantControl=Variant  PortDimensions=1
  Vel_min : Outport
  wires:
  Velocity/1 -> Vel_min/1

== system untitled2/HL Controller/Pos and Vel normalized1/Subsystem ==
  Angle : Inport
  In2 : Inport  Port=2
  Trigger : TriggerPort  VariantControl=Variant  PortDimensions=1
  Angle_min : Outport
  TS2R : Outport  Port=2
  wires:
  Angle/1 -> Angle_min/1
  In2/1 -> TS2R/1

== system untitled2/HL Controller/Pos and Vel normalized1/Subsystem1 ==
  Velocity : Inport
  Trigger : TriggerPort  VariantControl=Variant  PortDimensions=1
  Vel_max : Outport
  wires:
  Velocity/1 -> Vel_max/1

== system untitled2/HL Controller/Pos and Vel normalized1/Subsystem2 ==
  angle : Inport
  In2 : Inport  Port=2
  Trigger : TriggerPort  VariantControl=Variant  PortDimensions=1
  Angle_max : Outport
  TS1R : Outport  Port=2
  wires:
  angle/1 -> Angle_max/1
  In2/1 -> TS1R/1

== system untitled2/HL Controller/Pos and Vel normalized1/Subsystem3 ==
  Velocity : Inport
  Trigger : TriggerPort  VariantControl=Variant  PortDimensions=1
  Vel_min : Outport
  wires:
  Velocity/1 -> Vel_min/1

== system untitled2/HL Controller/STOP CONDITION BLOCK/LP filter ==
  x : Inport
  Constant : Constant  Value=2
  Integrator1 : Integrator  InitialConditionSource=external
  Integrator2 : Integrator
  Product : Product  RndMeth=Zero
  Product1 : Product  RndMeth=Zero
  Product2 : Product  Inputs=3  RndMeth=Zero
  Sum : Sum  Inputs=|+-
  Sum1 : Sum  Inputs=|+-
  wn : Constant  Value=wn
  x0 : Constant  Value=x0
  zt : Constant  Value=zt
  y : Outport  VectorParamsAs1DForOutWhenUnconnected=off
  yd : Outport  Port=2  VectorParamsAs1DForOutWhenUnconnected=off
  wires:
  Sum/1 -> Product/2
  wn/1 -> Product/1, Product1/1
  Sum1/1 -> Sum/1
  x0/1 -> Integrator1/2
  Integrator2/1 -> Product1/2, Product2/1
  Product/1 -> Integrator2/1
  x/1 -> Sum1/1
  Product1/1 -> Integrator1/1, yd/1
  Integrator1/1 -> Sum1/2, y/1
  Product2/1 -> Sum/2
  zt/1 -> Product2/3
  Constant/1 -> Product2/2

== system untitled2/HL Controller/STOP CONDITION BLOCK1/LP filter ==
  x : Inport
  Constant : Constant  Value=2
  Integrator1 : Integrator  InitialConditionSource=external
  Integrator2 : Integrator
  Product : Product  RndMeth=Zero
  Product1 : Product  RndMeth=Zero
  Product2 : Product  Inputs=3  RndMeth=Zero
  Sum : Sum  Inputs=|+-
  Sum1 : Sum  Inputs=|+-
  wn : Constant  Value=wn
  x0 : Constant  Value=x0
  zt : Constant  Value=zt
  y : Outport  VectorParamsAs1DForOutWhenUnconnected=off
  yd : Outport  Port=2  VectorParamsAs1DForOutWhenUnconnected=off
  wires:
  Sum/1 -> Product/2
  wn/1 -> Product/1, Product1/1
  Sum1/1 -> Sum/1
  x0/1 -> Integrator1/2
  Integrator2/1 -> Product1/2, Product2/1
  Product/1 -> Integrator2/1
  x/1 -> Sum1/1
  Product1/1 -> Integrator1/1, yd/1
  Integrator1/1 -> Sum1/2, y/1
  Product2/1 -> Sum/2
  zt/1 -> Product2/3
  Constant/1 -> Product2/2

== system untitled2/Initialize Function/Config_L /Enter Config Mode ==
  Compare To Zero8 : simulink/Logic and Bit Operations/Compare To Zero  relop===  OutDataTypeStr=boolean
  Constant5 : Constant  Value=0x00
  Start_Config_L : arduinolib/I2C Write  I2CModule=0  Mode=Master  SlaveAddress=0x28  SlaveByteOrder=BigEndian  Direction=Transmitter  RegisterAddressMode=on  RegisterAddress=0x3D  SlaveDataType=uint8  DataLength=1  NoAck=off  RepeatedStart=off  OutputStatus=on  blockPlatform=ARDUINO
      settings: SourceProductName=Common
  Status : Outport
  wires:
  Start_Config_L/1 -> Compare To Zero8/1  "0 for success"
  Constant5/1 -> Start_Config_L/1
  Compare To Zero8/1 -> Status/1

== system untitled2/Initialize Function/Config_L /Start Fused (NDOF) Mode ==
  Enable : EnablePort
  Compare To Constant2 : simulink/Logic and Bit Operations/Compare To Constant  relop===  const=0  OutDataTypeStr=boolean
  Constant4 : Constant  Value=0x0C
  I2C Write8 : arduinolib/I2C Write  I2CModule=0  Mode=Master  SlaveAddress=0x28  SlaveByteOrder=BigEndian  Direction=Transmitter  RegisterAddressMode=on  RegisterAddress=0x3D  SlaveDataType=uint8  DataLength=1  NoAck=off  RepeatedStart=off  OutputStatus=on  blockPlatform=ARDUINO
      settings: SourceProductName=Common
  Status : Outport
  wires:
  Compare To Constant2/1 -> Status/1
  Constant4/1 -> I2C Write8/1
  I2C Write8/1 -> Compare To Constant2/1  "0: success"

== system untitled2/Initialize Function/Config_L /X=Z, Y=Y, Z=X ==
  Enable : EnablePort
  Compare To Constant : simulink/Logic and Bit Operations/Compare To Constant  relop=~=  const=hex2dec('06')  OutDataTypeStr=boolean
  Compare To Constant1 : simulink/Logic and Bit Operations/Compare To Constant  relop===  const=hex2dec('06')  OutDataTypeStr=boolean
  Enabled Subsystem : Subsystem  TreatAsAtomicUnit=on
  I2C Read : arduinolib/I2C Read  I2CModule=0  Mode=Master  SlaveAddress=0x28  SlaveByteOrder=LittleEndian  Direction=Receiver  RegisterAddressMode=on  RegisterAddress=0x41  SlaveDataType=uint8  DataLength=1  NoAck=off  RepeatedStart=off  OutputStatus=off  blockPlatform=ARDUINO  SampleTime=-1
      settings: SourceProductName=Common
  OR : Logic  Operator=OR  IconShape=distinctive  AllPortsSameDT=off  OutDataTypeStr=boolean
  Status : Outport
  wires:
  I2C Read/1 -> Compare To Constant1/1, Compare To Constant/1
  Compare To Constant1/1 -> OR/2
  Compare To Constant/1 -> Enabled Subsystem/Enable
  Enabled Subsystem/1(Status) -> OR/1
  OR/1 -> Status/1
